simulink model "PID_control_for_a_quadrotor"  (R2016a)
settings: Solver=VariableStepAuto  StartTime=0.0  StopTime=10.0  RelTol=1e-3
settings Model: Creator=SRQ  LastModifiedBy=SRQ

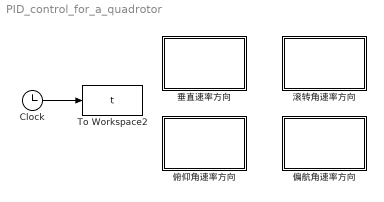
== system PID_control_for_a_quadrotor ==
  Clock : Clock
  To Workspace2 : ToWorkspace  VariableName=t  SampleTime=-1
  俯仰角速率方向 : Subsystem
  偏航角速率方向 : Subsystem
  垂直速率方向 : Subsystem
  滚转角速率方向 : Subsystem
  wires:
  Clock/1 -> To Workspace2/1

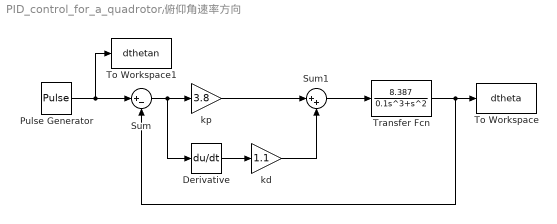
== system PID_control_for_a_quadrotor/俯仰角速率方向 ==
  Derivative : Derivative
  Pulse Generator : DiscretePulseGenerator  PulseType=Time based  Period=12  PulseWidth=25  PhaseDelay=3
  Sum : Sum  Inputs=|+-
  Sum1 : Sum  Inputs=|++
  To Workspace : ToWorkspace  VariableName=dtheta  SampleTime=-1
  To Workspace1 : ToWorkspace  VariableName=dthetan  SampleTime=-1
  Transfer Fcn : TransferFcn  Numerator=[8.387]  Denominator=[0.1 1 0 0]
  kd : Gain  Gain=1.1
  kp : Gain  Gain=3.8
  wires:
  Pulse Generator/1 -> To Workspace1/1, Sum/1
  Derivative/1 -> kd/1
  kp/1 -> Sum1/1
  Sum/1 -> Derivative/1, kp/1
  Transfer Fcn/1 -> Sum/2, To Workspace/1
  kd/1 -> Sum1/2
  Sum1/1 -> Transfer Fcn/1

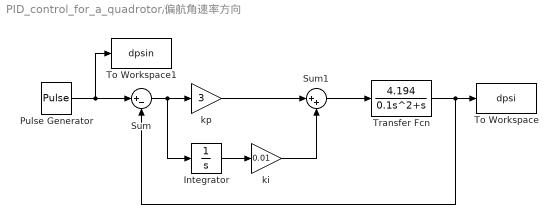
== system PID_control_for_a_quadrotor/偏航角速率方向 ==
  Integrator : Integrator
  Pulse Generator : DiscretePulseGenerator  PulseType=Time based  Period=12  PulseWidth=25  PhaseDelay=3
  Sum : Sum  Inputs=|+-
  Sum1 : Sum  Inputs=|++
  To Workspace : ToWorkspace  VariableName=dpsi  SampleTime=-1
  To Workspace1 : ToWorkspace  VariableName=dpsin  SampleTime=-1
  Transfer Fcn : TransferFcn  Numerator=[4.194]  Denominator=[0.1 1 0]
  ki : Gain  Gain=0.01
  kp : Gain  Gain=3
  wires:
  Pulse Generator/1 -> To Workspace1/1, Sum/1
  Integrator/1 -> ki/1
  kp/1 -> Sum1/1
  Sum/1 -> Integrator/1, kp/1
  Transfer Fcn/1 -> Sum/2, To Workspace/1
  ki/1 -> Sum1/2
  Sum1/1 -> Transfer Fcn/1

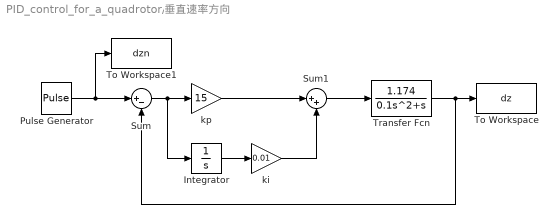
== system PID_control_for_a_quadrotor/垂直速率方向 ==
  Integrator : Integrator
  Pulse Generator : DiscretePulseGenerator  PulseType=Time based  Period=12  PulseWidth=25  PhaseDelay=3
  Sum : Sum  Inputs=|+-
  Sum1 : Sum  Inputs=|++
  To Workspace : ToWorkspace  VariableName=dz  SampleTime=-1
  To Workspace1 : ToWorkspace  VariableName=dzn  SampleTime=-1
  Transfer Fcn : TransferFcn  Numerator=[1.174]  Denominator=[0.1 1 0]
  ki : Gain  Gain=0.01
  kp : Gain  Gain=15
  wires:
  Pulse Generator/1 -> To Workspace1/1, Sum/1
  Integrator/1 -> ki/1
  kp/1 -> Sum1/1
  Sum/1 -> Integrator/1, kp/1
  Transfer Fcn/1 -> Sum/2, To Workspace/1
  ki/1 -> Sum1/2
  Sum1/1 -> Transfer Fcn/1

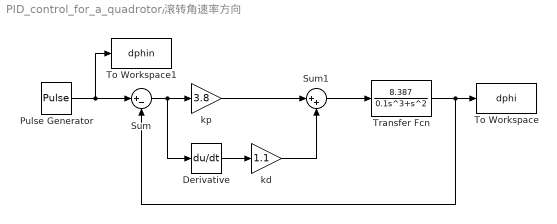
== system PID_control_for_a_quadrotor/滚转角速率方向 ==
  Derivative : Derivative
  Pulse Generator : DiscretePulseGenerator  PulseType=Time based  Period=12  PulseWidth=25  PhaseDelay=3
  Sum : Sum  Inputs=|+-
  Sum1 : Sum  Inputs=|++
  To Workspace : ToWorkspace  VariableName=dphi  SampleTime=-1
  To Workspace1 : ToWorkspace  VariableName=dphin  SampleTime=-1
  Transfer Fcn : TransferFcn  Numerator=[8.387]  Denominator=[0.1 1 0 0]
  kd : Gain  Gain=1.1
  kp : Gain  Gain=3.8
  wires:
  Pulse Generator/1 -> To Workspace1/1, Sum/1
  Derivative/1 -> kd/1
  kp/1 -> Sum1/1
  Sum/1 -> Derivative/1, kp/1
  Transfer Fcn/1 -> Sum/2, To Workspace/1
  kd/1 -> Sum1/2
  Sum1/1 -> Transfer Fcn/1
